simulink model "aula9_R2015"  (R2015a)
settings: Solver=ode3  StartTime=0.0  StopTime=5  RelTol=1e-3
values from neighbouring files (symbols this model uses):
  Ts = 0.05    [dados.mat]
undefined symbols (not defined in the file or in its folder): Dc, g2, K, K1, Nc, Ref, u0
libraries: simulink x1
settings Model: CovModelRefEnable=off  Creator=CBA2016-05  LastModifiedBy=CBA2016-05
settings DataIOCC: LimitDataPoints=off  SaveFormat=Dataset
settings HardwareCC: ProdBitPerPointer=64  ProdLargestAtomicFloat=Float  ProdIntDivRoundTo=Zero  ProdEndianess=LittleEndian  ProdHWDeviceType=Specified
settings ModelReferenceCC: PropagateSignalLabelsOutOfModel=on

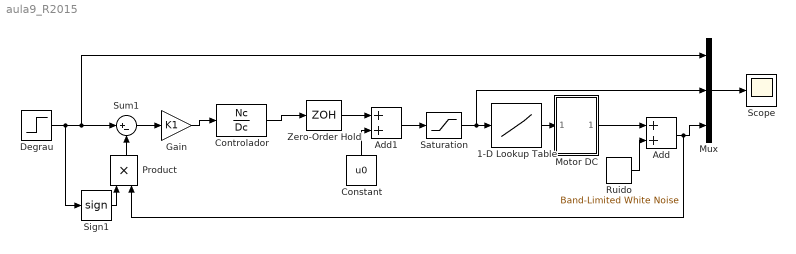
== system aula9_R2015 ==
  1-D Lookup Table : Lookup_n-D  NumberOfTableDimensions=1  BreakpointsForDimension1=[0,35,37,52,71,91,113,142,164,190,225]  Table=[0,0,330,850,1450,1930,2396,2793,3015,3224,3434]  InternalRulePriority=Speed  RndMeth=Simplest  InputSameDT=on
  Add : Sum
  Add1 : Sum
  Constant : Constant  Value=u0
  Controlador : TransferFcn  Numerator=Nc  Denominator=Dc
  Degrau : Step  Time=2  After=Ref  SampleTime=Ts
  Gain : Gain  Gain=K1
  "Motor DC " : Subsystem
  Mux : Mux  Inputs=3
  Product : Product
  Ruido : simulink/Sources/Band-Limited White Noise  Cov=0.1  Ts=Ts  seed=[23341]
  Saturation : Saturate  UpperLimit=256  LowerLimit=0
  Scope : Scope
      settings: TimeRange=auto  MaxDataPoints=5000  SaveName=X  YMin=-161.23409  YMax=1451.10682  SampleInput=on  SampleTime=Ts  DataFormat=Array
  Sign1 : Signum
  Sum1 : Sum  Inputs=|+-
  Zero-Order Hold : ZeroOrderHold  SampleTime=Ts
  wires:
  Mux/1 -> Scope/1
  Sum1/1 -> Gain/1
  Zero-Order Hold/1 -> Add1/1
  "Motor DC "/1(Out1) -> Add/1
  Ruido/1 -> Add/2
  Constant/1 -> Add1/2
  1-D Lookup Table/1 -> "Motor DC "/1(In1)
  Add1/1 -> Saturation/1
  Saturation/1 -> Mux/2, 1-D Lookup Table/1
  Add/1 -> Mux/3, Product/2
  Degrau/1 -> Sign1/1, Mux/1, Sum1/1
  Product/1 -> Sum1/2
  Sign1/1 -> Product/1
  Gain/1 -> Controlador/1
  Controlador/1 -> Zero-Order Hold/1

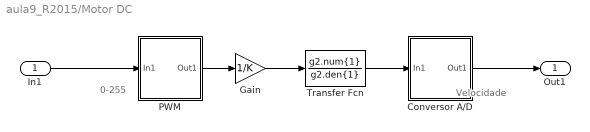
== system aula9_R2015/Motor DC  ==
  note: 0-255
  note: Velocidade
  In1 : Inport
  Conversor A/D : Subsystem
  Gain : Gain  Gain=1/K
  PWM : Subsystem
  Transfer Fcn : TransferFcn  Numerator=g2.num{1}  Denominator=g2.den{1}
  Out1 : Outport
  wires:
  Conversor A/D/1(Out1) -> Out1/1
  Transfer Fcn/1 -> Conversor A/D/1(In1)
  PWM/1(Out1) -> Gain/1
  In1/1 -> PWM/1(In1)
  Gain/1 -> Transfer Fcn/1

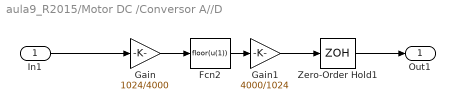
== system aula9_R2015/Motor DC /Conversor A//D ==
  In1 : Inport
  Fcn2 : Fcn  Expr=floor(u(1))
  Gain : Gain  Gain=1024/4000
  Gain1 : Gain  Gain=4000/1024
  Zero-Order Hold1 : ZeroOrderHold  SampleTime=Ts
  Out1 : Outport
  wires:
  Fcn2/1 -> Gain1/1
  Gain/1 -> Fcn2/1
  In1/1 -> Gain/1
  Zero-Order Hold1/1 -> Out1/1
  Gain1/1 -> Zero-Order Hold1/1

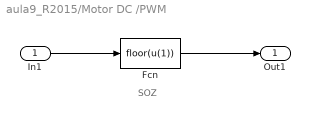
== system aula9_R2015/Motor DC /PWM ==
  note: SOZ
  In1 : Inport
  Fcn : Fcn  Expr=floor(u(1))
  Out1 : Outport
  wires:
  Fcn/1 -> Out1/1
  In1/1 -> Fcn/1
